simulink model "constrain_following_v3"  (R2024b)
settings: Solver=ode4  StartTime=0.0  StopTime=inf  FixedStep=1/20  MaxStep=5e-5  RelTol=1e-3
InitFcn:
  | init_controller;
undefined symbols (not defined in the file or in its folder): angular, cfcontroller, linear
libraries: ros2lib x4, simulink x2, sldrtlib x1
settings Model: Creator=Harry  LastModifiedBy=robot
settings SolverCC: ZeroCrossAlgorithm=Adaptive
settings DebuggingCC: UnconnectedInputMsg=warning  UnconnectedOutputMsg=warning  UnconnectedLineMsg=warning
settings ModelReferenceCC: EnableRefExpFcnMdlSchedulingChecks=on
settings RTWCC: GPUComputeCapability=3.5  DLArmComputeVersion=19.05

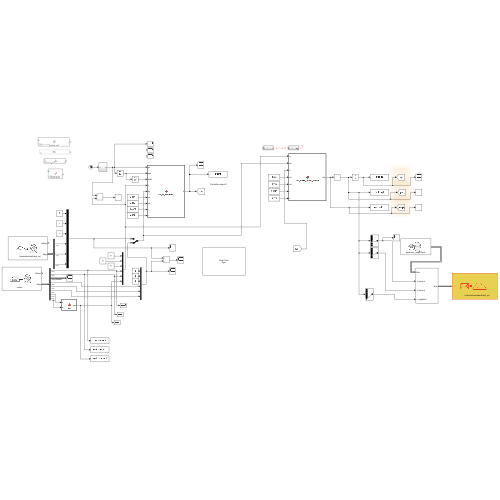
[thumbnail: Simulink's stored preview of the top-level diagram]
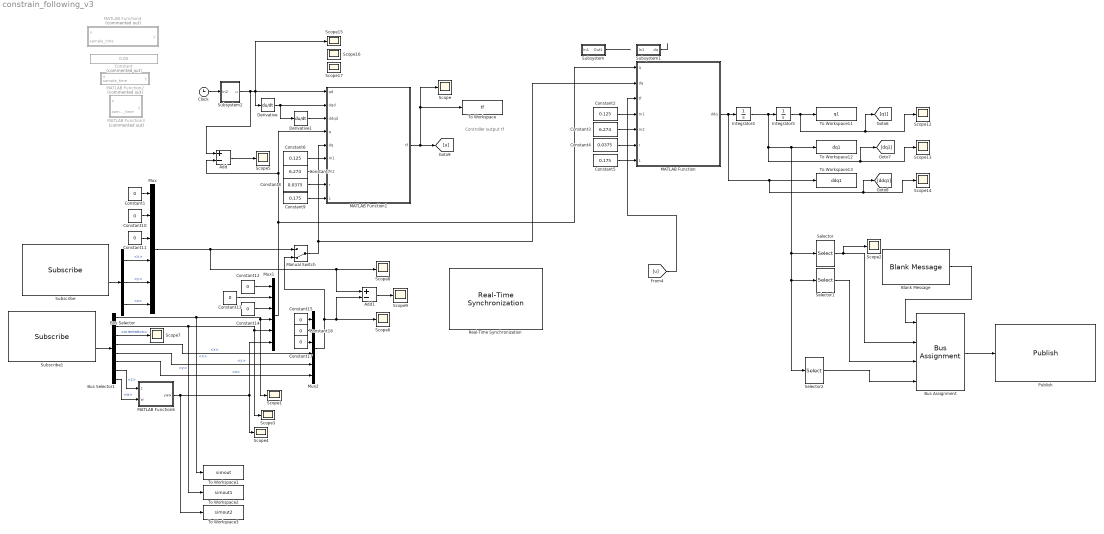
== system constrain_following_v3 ==
  note: Controller output tf
  Add : Sum  Inputs=+-
  Add1 : Sum  Inputs=+-
  Blank Message : ros2lib/Blank Message  messageClass=Message  entityType=geometry_msgs/Twist  messageType=geometry_msgs/Twist  SampleTime=inf
  Bus Assignment : BusAssignment  AssignedSignals=linear.x,linear.y,angular.z
  Bus Selector : BusSelector  OutputSignals=twist.twist.linear.x,twist.twist.linear.y,twist.twist.angular.z
  Bus Selector1 : BusSelector  OutputSignals=pose.pose.position.x,pose.pose.position.y,pose.pose.orientation,twist.twist.linear.x,twist.twist.linear.y,twist.twist.angular.z,pose.pose.orientation.z,pose.pose.orientation.w
  Clock : Clock
  Constant : Constant  Commented=on  Value=0.05
  Constant{1,10..17} (9 alike) : Constant  Value=0
  Constant2 : Constant  Value=0.125
  Constant3 : Constant  Value=6.274
  Constant4 : Constant  Value=0.0375
  Constant5 : Constant  Value=0.175
  Constant6 : Constant  Value=0.125
  Constant7 : Constant  Value=6.274
  Constant8 : Constant  Value=0.0375
  Constant9 : Constant  Value=0.175
  Derivative : Derivative
  Derivative1 : Derivative
  Integrator4 : Integrator  InitialCondition=[0;0;0;0;0;0]
  Integrator5 : Integrator  InitialCondition=[0;0;0;cfcontroller.init_x; cfcontroller.init_y; cfcontroller.init_theta]
  MATLAB Function : MATLAB Function  TreatAsAtomicUnit=on
  MATLAB Function1 : MATLAB Function  TreatAsAtomicUnit=on
  MATLAB Function2 : MATLAB Function  Commented=on  TreatAsAtomicUnit=on
  MATLAB Function3 : MATLAB Function  Commented=on  TreatAsAtomicUnit=on
  MATLAB Function4 : MATLAB Function  Commented=on  TreatAsAtomicUnit=on
  MATLAB Function6 : MATLAB Function  TreatAsAtomicUnit=on
  Manual Switch : ManualSwitch  CurrentSetting=0
  Mux : Mux  Inputs=6
  Mux1 : Mux  Inputs=6
  Mux2 : Mux  Inputs=6
  Publish : ros2lib/Publish  topicSource=Select from ROS network  topic=/chassis/command/cmd_vel  messageType=geometry_msgs/Twist  QOSHistory=Keep last  QOSDepth=1  QOSReliability=Best effort  QOSDurability=Volatile  QOSDeadline=Inf  QOSLifespan=Inf  QOSLiveliness=Automatic  QOSLeaseDuration=Inf  QOSAvoidROSNamespaceConventions=off
  Real-Time Synchronization : sldrtlib/Real-Time Synchronization  SampleTime=1/20  MaxMissedTicks=1000  ShowMissedTicks=off  YieldWhenWaiting=off
  Scope{,1..9,12..17} (16 alike) : Scope
  Selector : Selector  InputPortWidth=6  IndexOptions=Index vector (dialog)  Indices=4  OutputSizes=1
  Selector1 : Selector  InputPortWidth=6  IndexOptions=Index vector (dialog)  Indices=5  OutputSizes=1
  Selector2 : Selector  InputPortWidth=6  IndexOptions=Index vector (dialog)  Indices=6  OutputSizes=1
  Subscribe : ros2lib/Subscribe  topicSource=Specify your own  topic=/chassis/actual/cmd_vel  messageType=geometry_msgs/TwistWithCovarianceStamped  sampleTime=-1  QOSHistory=Keep last  QOSDepth=1  QOSReliability=Best effort  QOSDurability=Volatile  QOSDeadline=Inf  QOSLifespan=Inf  QOSLiveliness=Automatic  QOSLeaseDuration=Inf  QOSAvoidROSNamespaceConventions=off
  Subscribe1 : ros2lib/Subscribe  topicSource=Specify your own  topic=/odom  messageType=nav_msgs/Odometry  sampleTime=-1  QOSHistory=Keep last  QOSDepth=1  QOSReliability=Best effort  QOSDurability=Volatile  QOSDeadline=Inf  QOSLifespan=Inf  QOSLiveliness=Automatic  QOSLeaseDuration=Inf  QOSAvoidROSNamespaceConventions=off
  Subsystem : Subsystem
  Subsystem1 : Subsystem
  Subsystem2 : Subsystem
  To Workspace : ToWorkspace  VariableName=tf  SaveFormat=Timeseries  SampleTime=-1
  To Workspace1 : ToWorkspace  VariableName=simout  SaveFormat=Timeseries  SampleTime=-1
  To Workspace11 : ToWorkspace  VariableName=q1  SaveFormat=Timeseries  SampleTime=-1
  To Workspace12 : ToWorkspace  VariableName=dq1  SaveFormat=Timeseries  SampleTime=-1
  To Workspace13 : ToWorkspace  VariableName=ddq1  SaveFormat=Timeseries  SampleTime=-1
  To Workspace2 : ToWorkspace  VariableName=simout1  SaveFormat=Timeseries  SampleTime=-1
  To Workspace3 : ToWorkspace  VariableName=simout2  SaveFormat=Timeseries  SampleTime=-1
  wires:
  [u] -> MATLAB Function/3(tf)
  Constant2/1 -> MATLAB Function/4(m1)
  Constant3/1 -> MATLAB Function/5(m2)
  Constant4/1 -> MATLAB Function/6(r)
  Constant5/1 -> MATLAB Function/7(L)
  Integrator4/1 -> Scope13/1, [dq1], Selector2/1, Selector1/1, Selector/1, To Workspace12/1, Integrator5/1
  Integrator5/1 -> To Workspace11/1, [q1], Scope12/1
  MATLAB Function1/1(tf) -> To Workspace/1, Scope/1, [u]
  Constant6/1 -> MATLAB Function1/6(m1)
  Constant8/1 -> MATLAB Function1/8(r)
  Constant7/1 -> MATLAB Function1/7(m2)
  Constant9/1 -> MATLAB Function1/9(L)
  Subsystem2/1(u) -> Add/1, Derivative/1, Scope15/1, MATLAB Function1/1(qd)
  Subsystem/1(Out1) -> ?
  Subsystem1/1(dq) -> ?
  Clock/1 -> Subsystem2/1(In2)
  Derivative/1 -> Derivative1/1, MATLAB Function1/2(dqd)
  Derivative1/1 -> MATLAB Function1/3(ddqd)
  Subscribe/2 -> Bus Selector/1
  Constant10/1 -> Mux/2
  Constant11/1 -> Mux/3
  Bus Selector/1 -> Mux/4  "<x>"
  Bus Selector/2 -> Mux/5  "<y>"
  Bus Selector/3 -> Mux/6  "<z>"
  Constant1/1 -> Mux/1
  MATLAB Function/1(ddq) -> Scope14/1, [ddq1], To Workspace13/1, Integrator4/1
  Bus Assignment/1 -> Publish/1
  Blank Message/1 -> Bus Assignment/1
  Selector/1 -> Scope2/1, Bus Assignment/2
  Selector1/1 -> Bus Assignment/3
  Selector2/1 -> Bus Assignment/4
  Subscribe1/2 -> Bus Selector1/1
  Bus Selector1/3 -> Scope7/1  "<orientation>"
  Bus Selector1/4 -> Mux2/4  "<x>"
  Bus Selector1/5 -> Mux2/5  "<y>"
  Bus Selector1/6 -> Mux2/6  "<z>"
  Manual Switch/1 -> MATLAB Function/2(dq), MATLAB Function1/5(dq)
  Mux2/1 -> Manual Switch/2, Scope6/1, Add1/2
  Mux1/1 -> MATLAB Function/1(q), Add/2, MATLAB Function1/4(q)
  Mux/1 -> Add1/1, Scope8/1, Manual Switch/1
  Constant12/1 -> Mux1/1
  Constant13/1 -> Mux1/2
  Constant14/1 -> Mux1/3
  Bus Selector1/1 -> To Workspace1/1, Scope1/1, Mux1/4  "<x>"
  Bus Selector1/2 -> To Workspace2/1, Scope3/1, Mux1/5  "<y>"
  MATLAB Function6/1(yaw) -> To Workspace3/1, Mux1/6, Scope4/1
  Constant15/1 -> Mux2/1
  Constant16/1 -> Mux2/2
  Constant17/1 -> Mux2/3
  Add/1 -> Scope5/1
  Bus Selector1/7 -> MATLAB Function6/1(z)  "<z>"
  Bus Selector1/8 -> MATLAB Function6/2(w)  "<w>"
  Add1/1 -> Scope9/1

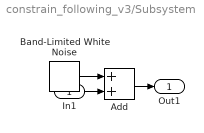
== system constrain_following_v3/Subsystem ==
  In1 : Inport
  Add : Sum
  Band-Limited White Noise : simulink/Sources/Band-Limited White Noise  Cov=[0.0001]  Ts=0.1  seed=[23341,23342,23343,23344,23345,23346]
  Out1 : Outport
  wires:
  Band-Limited White Noise/1 -> Add/1
  Add/1 -> Out1/1
  In1/1 -> Add/2

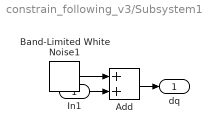
== system constrain_following_v3/Subsystem1 ==
  In1 : Inport
  Add : Sum
  Band-Limited White Noise1 : simulink/Sources/Band-Limited White Noise  Cov=[0.00001]  Ts=0.1  seed=[3341,3342,3343,3344,3345,3346]
  dq : Outport
  wires:
  Band-Limited White Noise1/1 -> Add/1
  Add/1 -> dq/1
  In1/1 -> Add/2

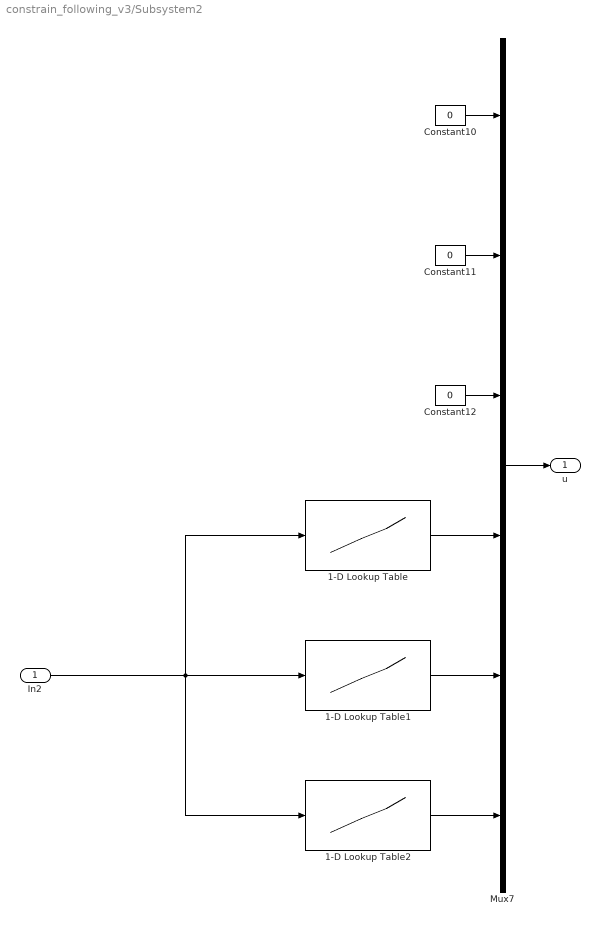
== system constrain_following_v3/Subsystem2 ==
  In2 : Inport
  1-D Lookup Table : Lookup_n-D  NumberOfTableDimensions=1  BreakpointsForDimension1=cfcontroller.tspan  Table=cfcontroller.x_design  InterpMethod=Akima spline  InternalRulePriority=Speed  RndMeth=Simplest
  1-D Lookup Table1 : Lookup_n-D  NumberOfTableDimensions=1  BreakpointsForDimension1=cfcontroller.tspan  Table=cfcontroller.y_design  InterpMethod=Akima spline  InternalRulePriority=Speed  RndMeth=Simplest
  1-D Lookup Table2 : Lookup_n-D  NumberOfTableDimensions=1  BreakpointsForDimension1=cfcontroller.tspan  Table=cfcontroller.theta_design  InterpMethod=Akima spline  InternalRulePriority=Speed  RndMeth=Simplest
  Constant10 : Constant  Value=0
  Constant11 : Constant  Value=0
  Constant12 : Constant  Value=0
  Mux7 : Mux  Inputs=6
  u : Outport
  wires:
  Mux7/1 -> u/1
  Constant10/1 -> Mux7/1
  Constant11/1 -> Mux7/2
  Constant12/1 -> Mux7/3
  1-D Lookup Table/1 -> Mux7/4
  1-D Lookup Table2/1 -> Mux7/6
  1-D Lookup Table1/1 -> Mux7/5
  In2/1 -> 1-D Lookup Table2/1, 1-D Lookup Table/1, 1-D Lookup Table1/1

== matlab function constrain_following_v3/MATLAB Function1 ==
  data: qd input; dqd input; ddqd input; q input; tf output; dq input; m1 input; m2 input; r input; L input
function tf = run_cf_controller(qd, dqd, ddqd, q, dq, m1, m2, r, L)
    qd   = reshape(qd, [6,1]);
    dqd  = reshape(dqd,[6,1]);
    ddqd = reshape(ddqd,[6,1]);
    q    = reshape(q, [6,1]);
    dq   = reshape(dq,[6,1]);
    tf   = cf_controller(qd, dqd, ddqd, q, dq, m1, m2, r, L);

== matlab function constrain_following_v3/MATLAB Function ==
  data: q input; ddq output; dq input; tf input; m1 input; m2 input; r input; L input
function ddq = run_omni_robot_model(q, dq, tf, m1, m2, r, L)
    q  = reshape(q, [6,1]);
    dq = reshape(dq,[6,1]);
    tf = reshape(tf,[3,1]);
    ddq = omni_robot_model(q, dq, tf, m1, m2, r, L);

== matlab function constrain_following_v3/MATLAB Function4 ==
  settings: updateMethod=DISCRETE
  data: u input; y output; sample_time input
function y = derivative2(u, sample_time)
    %% 使用持久变量保存
    persistent u_1 u_2 u_3 index
    if isempty(u_1)
        u_1 = [0;0;0;0;0;0];
        u_2 = [0;0;0;0;0;0];
        u_3 = [0;0;0;0;0;0];
        index = 0;
    end
    index = index + 1;

    %% 输出数值导数
    sample_time2 = sample_time*sample_time;
    if index == 1
        y = [0;0;0;0;0;0];
    elseif index == 2
        y = [0;0;0;0;0;0];
    elseif index == 3
        y = (u_2 - 2*u_1 + u)/sample_time2;
    else
        y = (-1*u_3 + 4*u_2 - 5*u_1 + 2*u)/sample_time2;
    end

    %% 保存变量
    u_3 = u_2;
    u_2 = u_1;
    u_1 = u;
end

== matlab function constrain_following_v3/MATLAB Function3 ==
  settings: updateMethod=DISCRETE
  data: u input; y output; sample_time input
function y = derivative(u, sample_time)
    %% 使用持久变量保存
    persistent u_1 u_2 index
    if isempty(u_1)
        u_1 = [0;0;0;0;0;0];
        u_2 = [0;0;0;0;0;0];
        index = 0;
    end
    index = index + 1;

    %% 输出数值导数
    if index == 1
        y = [0;0;0;0;0;0];
    elseif index == 2
        y = (-u_1 + u)/sample_time;
    else
        y = (1*u_2 - 4*u_1 + 3*u)/(sample_time*2);
    end

    %% 保存变量

    u_2 = u_1;
    u_1 = u;
end

== matlab function constrain_following_v3/MATLAB Function6 ==
  data: z input; yaw output; w input
function yaw = fcn(z,w)
    % 声明输出大小和类型
    yaw = 0.0;  % 初始化为标量double类型
    
    
    yaw = atan2(2*w*z, 1 - 2*z*z);

== matlab function constrain_following_v3/MATLAB Function2 ==
  settings: updateMethod=DISCRETE  sampleTime=RateAngleControl
  data: u input; y output; sample_time input
function y = derivative(u, sample_time)
    %% 使用持久变量保存
    persistent u_1 u_2 index
    if isempty(u_1)
        u_1 = 0;
        u_2 = 0;
        index = 0;
    end
    index = index + 1;

    %% 输出数值导数
    if index == 1
        y = 0;
    elseif index == 2
        y = (-u_1 + u)/sample_time;
    else
        y = (1*u_2 - 4*u_1 + 3*u)/(sample_time*2);
    end

    %% 保存变量

    u_2 = u_1;
    u_1 = u;
end
